simulink model "fuzzy_hw3"  (R2018a)
settings: Solver=VariableStepAuto  StartTime=0.0  StopTime=10.0  RelTol=1e-3
libraries: fuzblock x1, simulink x1
settings Model: Creator=Danial  LastModifiedBy=Danial
settings DataIOCC: ReturnWorkspaceOutputs=on
settings SFSimCC: SimUseLocalCustomCode=on
settings RTWCC: RTWUseLocalCustomCode=on

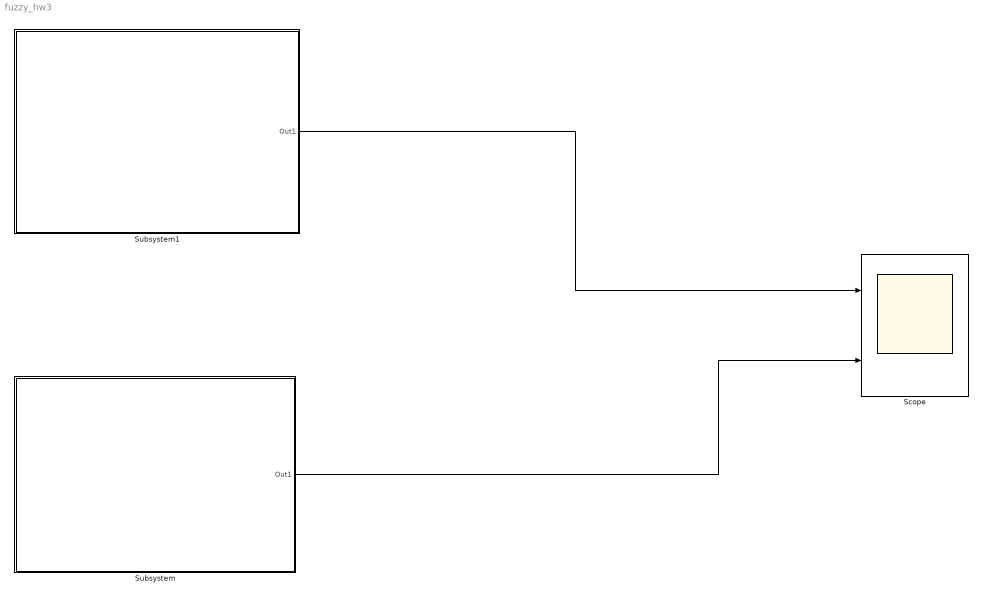
== system fuzzy_hw3 ==
  Scope : Scope  NumInputPorts=2
  Subsystem : Subsystem
  Subsystem1 : Subsystem
  wires:
  Subsystem1/1(Out1) -> Scope/1
  Subsystem/1(Out1) -> Scope/2

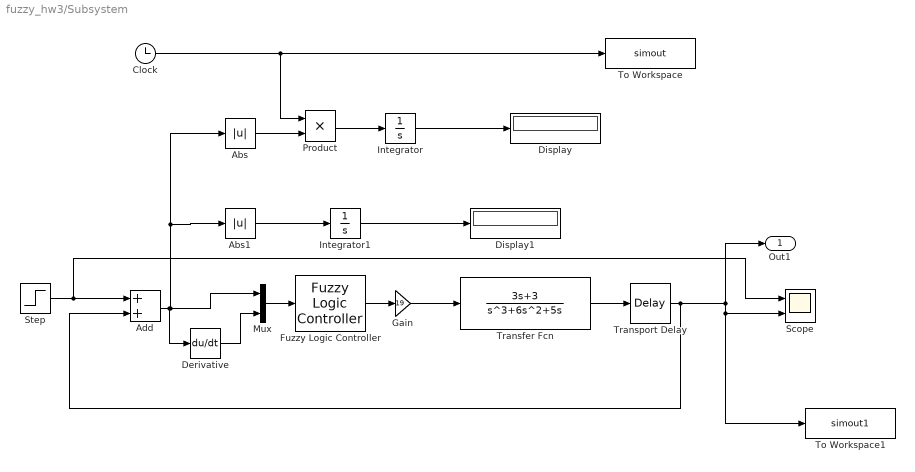
== system fuzzy_hw3/Subsystem ==
  Abs : Abs
  Abs1 : Abs
  Add : Sum
  Clock : Clock
  Derivative : Derivative
  Display : Display
  Display1 : Display
  Fuzzy Logic Controller : fuzblock/Fuzzy Logic  Controller  FIS=fuzzy_hw1  OutputSampleNumber=101  DataType=double  FuzzifiedInputs=off  RuleFiringStrengths=off  RuleOutputs=off  AggregatedOutputs=off  SimulateUsing=Interpreted execution  OutOfRangeInputValueMessage=warning  NoRuleFiredMessage=warning  EmptyOutputFuzzySetMessage=warning
  Gain : Gain  Gain=19
  Integrator : Integrator
  Integrator1 : Integrator
  Mux : Mux  Inputs=2
  Product : Product
  Scope : Scope  NumInputPorts=2
  Step : Step  SampleTime=0
  To Workspace : ToWorkspace  VariableName=simout  SaveFormat=Timeseries  SampleTime=-1
  To Workspace1 : ToWorkspace  VariableName=simout1  SaveFormat=Timeseries  SampleTime=-1
  Transfer Fcn : TransferFcn  Numerator=[3 3]  Denominator=[1 6 5 0]
  Transport Delay : TransportDelay
  Out1 : Outport
  wires:
  Add/1 -> Abs1/1, Abs/1, Mux/1, Derivative/1
  Transport Delay/1 -> To Workspace1/1, Scope/2, Out1/1, Add/2
  Clock/1 -> To Workspace/1, Product/1
  Integrator/1 -> Display/1
  Gain/1 -> Transfer Fcn/1
  Derivative/1 -> Mux/2
  Product/1 -> Integrator/1
  Transfer Fcn/1 -> Transport Delay/1
  Integrator1/1 -> Display1/1
  Abs/1 -> Product/2
  Abs1/1 -> Integrator1/1
  Step/1 -> Scope/1, Add/1
  Mux/1 -> Fuzzy Logic Controller/1
  Fuzzy Logic Controller/1 -> Gain/1

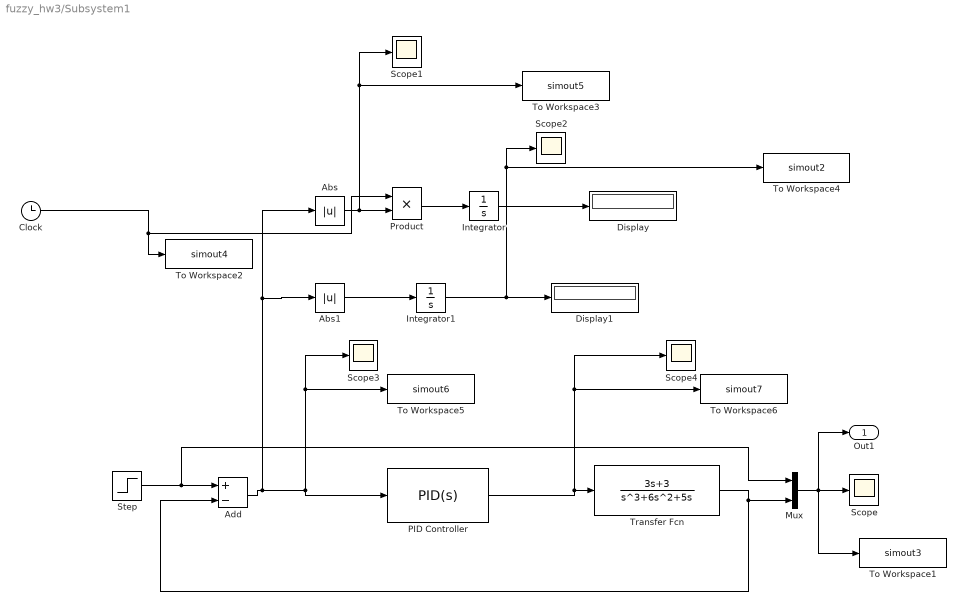
== system fuzzy_hw3/Subsystem1 ==
  Abs : Abs
  Abs1 : Abs
  Add : Sum  Inputs=+-
  Clock : Clock
  Display : Display
  Display1 : Display
  Integrator : Integrator
  Integrator1 : Integrator
  Mux : Mux  Inputs=2
  PID Controller : simulink/Continuous/PID Controller  Controller=PID  Form=Parallel  TimeDomain=Continuous-time  SampleTime=-1  IntegratorMethod=Forward Euler  FilterMethod=Forward Euler  ControllerParametersSource=internal  P=30  I=21.2  D=9  UseFilter=on  N=1  TunerSelectOption=Transfer Function Based (PID Tuner App)  InitialConditionSource=internal  InitialConditionForIntegrator=0  InitialConditionForFilter=0  DifferentiatorICPrevScaledInput=0  ExternalReset=none  TrackingMode=off  Kt=1  LimitOutput=off  UpperSaturationLimit=inf  LowerSaturationLimit=-inf  LinearizeAsGain=on  AntiWindupMode=none  Kb=1  POutMin=[]  POutMax=[]  IOutMin=[]  IOutMax=[]  DOutMin=[]  DOutMax=[]  NOutMin=[]  NOutMax=[]  SumOutMin=[]  SumOutMax=[]  SaturationOutMin=[]  SaturationOutMax=[]  PParamMin=[]  PParamMax=[]  IParamMin=[]  IParamMax=[]  DParamMin=[]  DParamMax=[]  NParamMin=[]  NParamMax=[]  KbParamMin=[]  KbParamMax=[]  KtParamMin=[]  KtParamMax=[]  KbOutMin=[]  KbOutMax=[]  KtOutMin=[]  KtOutMax=[]  IntegratorOutMin=[]  IntegratorOutMax=[]  FilterOutMin=[]  FilterOutMax=[]  SumI1OutMin=[]  SumI1OutMax=[]  SumI2OutMin=[]  SumI2OutMax=[]  SumI3OutMin=[]  SumI3OutMax=[]  SumDOutMin=[]  SumDOutMax=[]  DifferentiatorOutMin=[]  DifferentiatorOutMax=[]  FilterDiffOutCoefMin=[]  FilterDiffOutCoefMax=[]  ReciprocalOutMin=[]  ReciprocalOutMax=[]  SumDenOutMin=[]  SumDenOutMax=[]  SumNumOutMin=[]  SumNumOutMax=[]  DivideOutMin=[]  DivideOutMax=[]  IntegratorContinuousStateAttributes=''  IntegratorStateMustResolveToSignalObject=off  IntegratorRTWStateStorageClass=Auto  FilterContinuousStateAttributes=''  FilterStateMustResolveToSignalObject=off  FilterRTWStateStorageClass=Auto
  Product : Product
  Scope{,1..4} (5 alike) : Scope
  Step : Step  SampleTime=0
  To Workspace1 : ToWorkspace  VariableName=simout3  SaveFormat=Timeseries  SampleTime=-1
  To Workspace2 : ToWorkspace  VariableName=simout4  SaveFormat=Timeseries  SampleTime=-1
  To Workspace3 : ToWorkspace  VariableName=simout5  SaveFormat=Timeseries  SampleTime=-1
  To Workspace4 : ToWorkspace  VariableName=simout2  SaveFormat=Timeseries  SampleTime=-1
  To Workspace5 : ToWorkspace  VariableName=simout6  SaveFormat=Timeseries  SampleTime=-1
  To Workspace6 : ToWorkspace  VariableName=simout7  SaveFormat=Timeseries  SampleTime=-1
  Transfer Fcn : TransferFcn  Numerator=[3 3]  Denominator=[1 6 5 0]
  Out1 : Outport
  wires:
  Abs/1 -> Product/2, To Workspace3/1, Scope1/1
  Step/1 -> Mux/1, Add/1
  Transfer Fcn/1 -> Add/2, Mux/2
  Add/1 -> To Workspace5/1, Scope3/1, PID Controller/1, Abs1/1, Abs/1
  Integrator1/1 -> To Workspace4/1, Scope2/1, Display1/1
  Clock/1 -> To Workspace2/1, Product/1
  Mux/1 -> Out1/1, To Workspace1/1, Scope/1
  Abs1/1 -> Integrator1/1
  PID Controller/1 -> To Workspace6/1, Scope4/1, Transfer Fcn/1
  Product/1 -> Integrator/1
  Integrator/1 -> Display/1
